simulink model "Final_Q6"  (R2020a)
settings: Solver=VariableStepAuto  StartTime=0.0  StopTime=10.0  RelTol=1e-3
values from neighbouring files (symbols this model uses):
  PDden = [1 932.093]    [Final_Q6.m]
  PDnum = [457215 456725]    [Final_Q6.m]
  PIden = [1 0]    [Final_Q6.m]
  PInum = [52.6 52.6]    [Final_Q6.m]
  TsD = 0.002    [Final_Q6.m]
  TsI = 0.2    [Final_Q6.m]
settings Model: Creator=Joey Baby  LastModifiedBy=Joey Baby

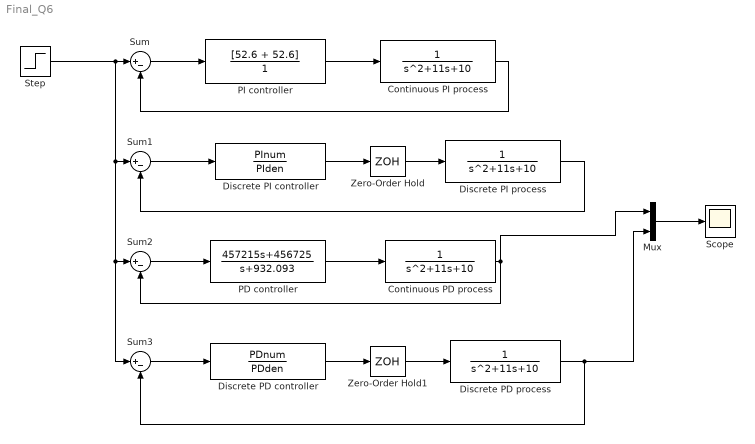
== system Final_Q6 ==
  Continuous PD process : TransferFcn  Denominator=[1 11 10]
  Continuous PI process : TransferFcn  Denominator=[1 11 10]
  Discrete PI controller : DiscreteTransferFcn  Numerator=PInum  Denominator=PIden  SampleTime=TsI
  "Discrete PD controller " : DiscreteTransferFcn  Numerator=PDnum  Denominator=PDden  SampleTime=TsD
  Discrete PD process : TransferFcn  Denominator=[1 11 10]
  Discrete PI process : TransferFcn  Denominator=[1 11 10]
  Mux : Mux  Inputs=2
  PD controller : TransferFcn  Numerator=[457215 456725]  Denominator=[1 932.093]
  PI controller : TransferFcn  Numerator=[52.6 + 52.6]  Denominator=[1]
  Scope : Scope
  Step : Step  SampleTime=0
  Sum{,1..3} (4 alike) : Sum  Inputs=|+-
  Zero-Order Hold : ZeroOrderHold  SampleTime=TsI
  Zero-Order Hold1 : ZeroOrderHold  SampleTime=TsD
  wires:
  Step/1 -> Sum3/1, Sum2/1, Sum1/1, Sum/1
  Sum/1 -> PI controller/1
  PI controller/1 -> Continuous PI process/1
  Continuous PI process/1 -> Sum/2
  Sum1/1 -> Discrete PI controller/1
  Discrete PI controller/1 -> Zero-Order Hold/1
  Zero-Order Hold/1 -> Discrete PI process/1
  Discrete PI process/1 -> Sum1/2
  PD controller/1 -> Continuous PD process/1
  Sum2/1 -> PD controller/1
  Continuous PD process/1 -> Mux/1, Sum2/2
  Sum3/1 -> "Discrete PD controller "/1
  "Discrete PD controller "/1 -> Zero-Order Hold1/1
  Zero-Order Hold1/1 -> Discrete PD process/1
  Discrete PD process/1 -> Mux/2, Sum3/2
  Mux/1 -> Scope/1
